simulink model "cp_lambda"  (R2024a)
settings: Solver=VariableStepAuto  StartTime=0.0  StopTime=20  RelTol=1e-3
values from neighbouring files (symbols this model uses):
  cp = [1e-05 1e-05 1e-05 1e-05 1e-05 1e-05 1e-05 1e-05 1e-05 1e-05 1e-05 1e-05 ... (3015 elements, 15x201)]    [CP.mat]
  pitch = [1 3 5 7 9 11 13 15 17 19 21 23 ... (15 elements, 1x15)]    [CP.mat]
  TSR = [0 0.1 0.2 0.3 0.4 0.5 0.6 0.7 0.8 0.9 1 1.1 ... (201 elements, 1x201)]    [CP.mat]
libraries: simulink x5
settings Model: Creator=emanuele  LastModifiedBy=emanuele

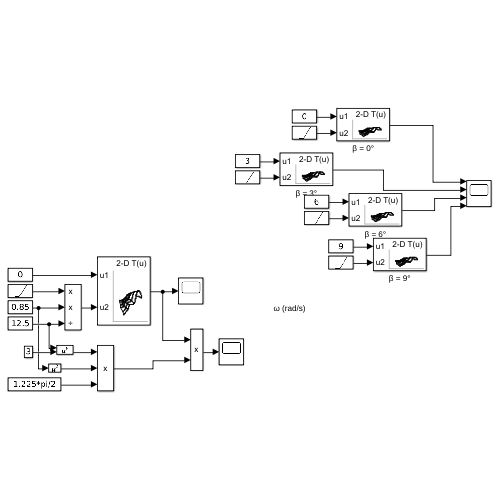
[thumbnail: Simulink's stored preview of the top-level diagram]
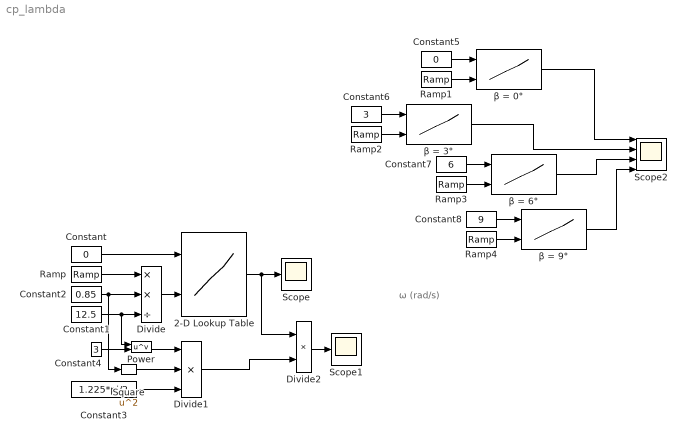
== system cp_lambda ==
  note: ω (rad/s)
  2-D Lookup Table : Lookup_n-D  BreakpointsForDimension1=pitch  BreakpointsForDimension2=TSR  Table=cp  InterpMethod=Cubic spline  InternalRulePriority=Speed  RndMeth=Simplest
      settings: InputPortMap=u0,u1
  Constant : Constant  Value=0
  Constant1 : Constant  Value=12.5
  Constant2 : Constant  Value=0.85
  Constant3 : Constant  Value=1.225*pi/2
  Constant4 : Constant  Value=3
  Constant5 : Constant  Value=0
  Constant6 : Constant  Value=3
  Constant7 : Constant  Value=6
  Constant8 : Constant  Value=9
  Divide : Product  Inputs=**/
  Divide1 : Product  Inputs=***
  Divide2 : Product
  Power : Math  Operator=pow
  Ramp{,1..4} (5 alike) : simulink/Sources/Ramp  slope=1  start=0  InitialOutput=0
  Scope : Scope
  Scope1 : Scope
  Scope2 : Scope  NumInputPorts=4
  Square : Math  Operator=square
  β = 0° : Lookup_n-D  BreakpointsForDimension1=pitch  BreakpointsForDimension2=TSR  Table=cp  InterpMethod=Cubic spline  InternalRulePriority=Speed  RndMeth=Simplest
      settings: InputPortMap=u0,u1
  β = 3° : Lookup_n-D  BreakpointsForDimension1=pitch  BreakpointsForDimension2=TSR  Table=cp  InterpMethod=Cubic spline  InternalRulePriority=Speed  RndMeth=Simplest
      settings: InputPortMap=u0,u1
  β = 6° : Lookup_n-D  BreakpointsForDimension1=pitch  BreakpointsForDimension2=TSR  Table=cp  InterpMethod=Cubic spline  InternalRulePriority=Speed  RndMeth=Simplest
      settings: InputPortMap=u0,u1
  β = 9° : Lookup_n-D  BreakpointsForDimension1=pitch  BreakpointsForDimension2=TSR  Table=cp  InterpMethod=Cubic spline  InternalRulePriority=Speed  RndMeth=Simplest
      settings: InputPortMap=u0,u1
  wires:
  Constant/1 -> 2-D Lookup Table/1
  2-D Lookup Table/1 -> Divide2/1, Scope/1
  Constant1/1 -> Power/1, Divide/3
  Ramp/1 -> Divide/1
  Constant2/1 -> Square/1, Divide/2
  Divide/1 -> 2-D Lookup Table/2
  Constant3/1 -> Divide1/3
  Square/1 -> Divide1/2
  Power/1 -> Divide1/1
  Constant4/1 -> Power/2
  Divide2/1 -> Scope1/1
  Divide1/1 -> Divide2/2
  β = 0°/1 -> Scope2/1
  Constant5/1 -> β = 0°/1
  Ramp1/1 -> β = 0°/2
  Ramp2/1 -> β = 3°/2
  Constant6/1 -> β = 3°/1
  Constant7/1 -> β = 6°/1
  Ramp3/1 -> β = 6°/2
  Ramp4/1 -> β = 9°/2
  Constant8/1 -> β = 9°/1
  β = 3°/1 -> Scope2/2
  β = 6°/1 -> Scope2/3
  β = 9°/1 -> Scope2/4
